simulink model "blockdemo"  (Simulink 6.3)
settings: Solver=FixedStepDiscrete  StartTime=0.0  StopTime=20.0  RelTol=1e-3
InitFcn:
  | %% DSPBuilder Start
  | alt_dspbuilder_update_model(bdroot)
  | %% DSPBuilder End
libraries: allblocks_alteradspbuilder2 x8
settings Model: Creator=cpurcell  LastModifiedBy=delphick
settings DebuggingCC: MultiTaskDSMMsg=error

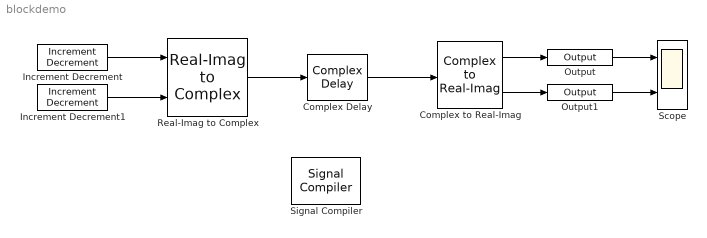
== system blockdemo ==
  Complex Delay : allblocks_alteradspbuilder2/Complex Delay  pipeline=10  ClockPhase=1  use_ena=off  use_sclr=off
  Complex to Real-Imag : allblocks_alteradspbuilder2/Complex to Real-Imag  BusType=Signed Integer  bwl=4  bwr=0
  Increment Decrement : allblocks_alteradspbuilder2/Increment Decrement  BusType=Signed Integer  bwl=4  bwr=8  SpecifyClock=off  clr_value=0  direction=Increment  phase_selection=1  use_ena=off  use_sclr=off
  Increment Decrement1 : allblocks_alteradspbuilder2/Increment Decrement  BusType=Signed Integer  bwl=4  bwr=8  SpecifyClock=off  clr_value=8  direction=Increment  phase_selection=1  use_ena=off  use_sclr=off
  Output : allblocks_alteradspbuilder2/Output  iofile=C:\workspace_clean\Documentation\DesignExamples\Tutorials\UnitBlocks\Complex\ComplexDelay\tb_blockdemo\blockdemo_Output.capture  BusType=Inferred  bwl=8  bwr=0  PORTTYPE=Output
  Output1 : allblocks_alteradspbuilder2/Output  iofile=C:\workspace_clean\Documentation\DesignExamples\Tutorials\UnitBlocks\Complex\ComplexDelay\tb_blockdemo\blockdemo_Output1.capture  BusType=Inferred  bwl=8  bwr=0  PORTTYPE=Output
  Real-Imag to Complex : allblocks_alteradspbuilder2/Real-Imag to Complex  BusType=Signed Integer  bwl=4  bwr=0
  Scope : Scope  NumInputPorts=2
      settings: TimeRange=20  YMin=-10~-10  YMax=10~10
  Signal Compiler : allblocks_alteradspbuilder2/Signal Compiler  DeviceFamily=Stratix IV  DeviceName=AUTO  EnableSignalTap=off  SignalTapDepth=128  UseBoardBlock=off  StpUseDefaultClock=on  StpClock=clock
  wires:
  Complex to Real-Imag/1 -> Output/1
  Complex to Real-Imag/2 -> Output1/1
  Output/1 -> Scope/1
  Output1/1 -> Scope/2
  Increment Decrement/1 -> Real-Imag to Complex/1
  Increment Decrement1/1 -> Real-Imag to Complex/2
  Real-Imag to Complex/1 -> Complex Delay/1
  Complex Delay/1 -> Complex to Real-Imag/1
